simulink model "twotwothree999"  (R2013b)
settings: Solver=ode3  StartTime=0.01  StopTime=50  FixedStep=0.001  RelTol=1e-3
libraries: simulink x2
settings Model: Creator=TheWhitescar  LastModifiedBy=286
settings DebuggingCC: MultiTaskDSMMsg=warning  MultiTaskCondExecSysMsg=none  FcnCallInpInsideContextMsg=EnableAllAsWarning
settings RTWCC: IncludeERTFirstTime=on

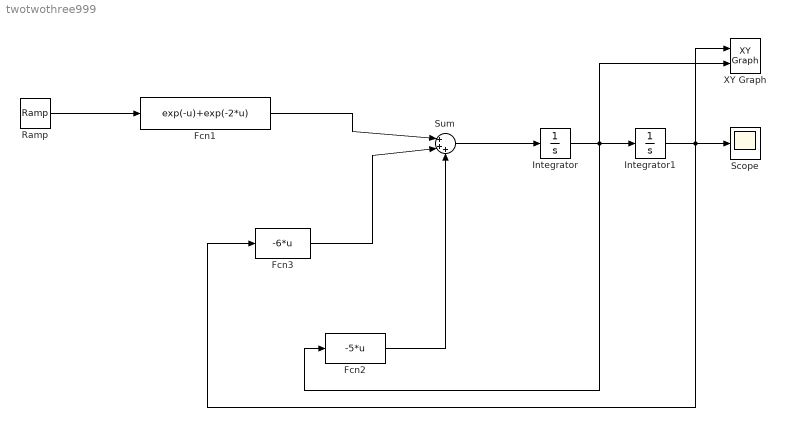
== system twotwothree999 ==
  Fcn1 : Fcn  Expr=exp(-u)+exp(-2*u)
  Fcn2 : Fcn  Expr=-5*u
  Fcn3 : Fcn  Expr=-6*u
  Integrator : Integrator
  Integrator1 : Integrator
  Ramp : simulink/Sources/Ramp  slope=1  start=0  X0=0
  Scope : Scope
  Sum : Sum  Inputs=|+++
  XY Graph : simulink/Sinks/XY Graph  xmin=-1  xmax=1  ymin=-1  ymax=1  st=-1
  wires:
  Fcn1/1 -> Sum/1
  Fcn3/1 -> Sum/2
  Fcn2/1 -> Sum/3
  Sum/1 -> Integrator/1
  Integrator/1 -> Fcn2/1, XY Graph/2, Integrator1/1
  Integrator1/1 -> Fcn3/1, XY Graph/1, Scope/1
  Ramp/1 -> Fcn1/1
